simulink model "TS_example"  (Simulink 7.4)
settings: Solver=ode45  StartTime=0.0  StopTime=100.0  RelTol=1e-3
libraries: vrlib x2
settings Model: Creator=bgovinda  LastModifiedBy=bgovinda

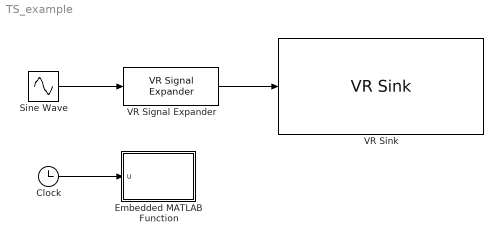
== system TS_example ==
  Clock : Clock
      settings: Decimation=10
  Embedded MATLAB Function : Stateflow chart
  Sine Wave : Sin  Amplitude=1  Bias=0  Frequency=1  Phase=0  Samples=10  SampleTime=0  Offset=0
  VR Signal Expander : vrlib/VR Signal Expander  SystemSampleTime=-1  outwidth=3  outidx=[2 3]
  VR Sink : vrlib/VR Sink  InstantiateOnLoad=on  SampleTime=0.1  ViewEnable=on  RemoteChange=off  RemoteView=off  FieldsWritten=Material2.emissiveColor.3.1.double  WorldFileName=example.wrl  AutoView=off  VideoDimensions=[]  FigureProperties="{'Position', 'Name', 'Viewpoint', 'CameraBound', 'CameraDirection', 'CameraPosition', 'CameraUpVector', 'ZoomFactor', 'Antialiasing', 'Headlight', 'Lighting', 'NavPanel', 'StatusBar', 'ToolBar', 'Textures', 'Transparency', 'Wireframe', 'NavZones', 'NavMode', 'NavSpeed', 'Record2DCompressMethod', 'Record2DCompressQuality', 'Record2D', 'Record2DFileName', 'Record2DFPS'; [5.0000000000000000e+000  9.2000000000000000e+001  5.7600000000000000e+002  3.8000000000000000e+002], '', '_untitled_2', 'on', [0.0000000000000000e+000  0.0000000000000000e+000 -1.0000000000000000e+000], [0.0000000000000000e+000  0.0000000000000000e+000  0.0000000000000000e+000], [0.0000000000000000e+000  1.0000000000000000e+000  0.0000000000000000e+000], [1.0000000000000000e+000], 'off', 'on', 'on', 'halfbar', 'on', 'on', 'on', 'on', 'off', 'off', 'fly', 'normal', 'auto', [7.5000000000000000e+001], 'off', '%f_anim_%n.avi', [1.5000000000000000e+001]}"
  wires:
  Sine Wave/1 -> VR Signal Expander/1
  VR Signal Expander/1 -> VR Sink/1
  Clock/1 -> Embedded MATLAB Function/1(u)

== matlab function Embedded MATLAB Function ==
  data: u input double
function fcn(u)
%#eml
eml.extrinsic('vrgcf');

persistent t;

if isempty(t)
    t = -1;
end

if (~mod(u,10))
    if (t==1)
        f=vrgcf;
        set(f,'Viewpoint','Viewpoint2');
        t = -1;
    else
        f=vrgcf;
        set(f,'Viewpoint','Viewpoint1');
        t = 1;
    end
end
